simulink model "MPC_Quad_4SV"  (R2022b)
settings: Solver=FixedStepAuto  StartTime=0.0  StopTime=250  FixedStep=Ts  RelTol=1e-3
undefined symbols (not defined in the file): A, B, C, Cm, Ct, D, estim_hover_nrpm, g, initState, Ir, Ixx, Iyy, Izz, Length, mass
libraries: sharedtransform x5, uavutilslib x2, mpclib x1, shared6dof x1, aerolibutil x1
settings Model: PacingRate=0.005000  Creator=Bw Jiang  LastModifiedBy=Bw Jiang
settings DebuggingCC: AlgebraicLoopMsg=none  ParameterOverflowMsg=none  ParameterUnderflowMsg=error

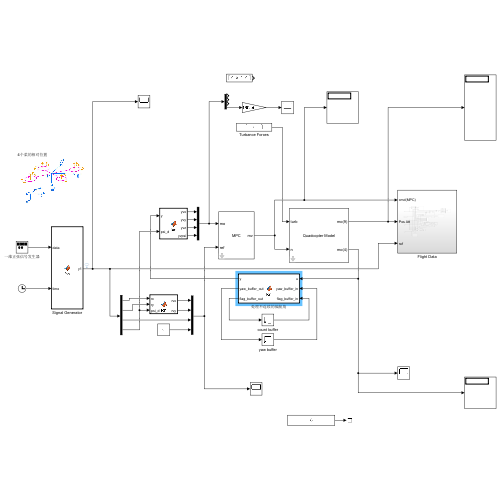
[thumbnail: Simulink's stored preview of the top-level diagram]
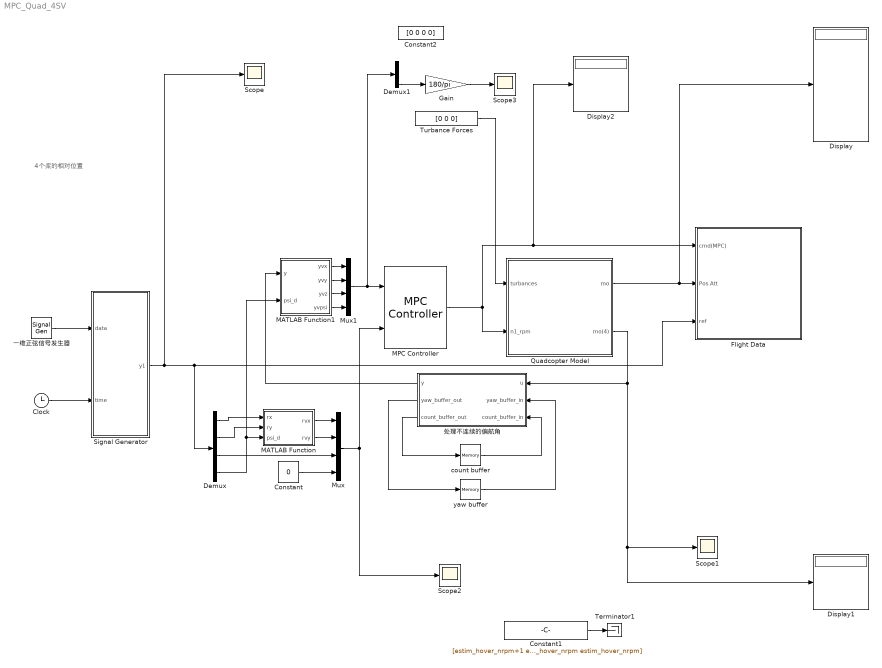
== system MPC_Quad_4SV ==
  note: 4个桨的相对位置
  Clock : Clock
  Constant : Constant  Value=0
  Constant1 : Constant  Value=[estim_hover_nrpm+1 estim_hover_nrpm estim_hover_nrpm estim_hover_nrpm]
  Constant2 : Constant  Value=[0 0 0 0]
  Demux : Demux
  Demux1 : Demux
  Display : Display
  Display1 : Display
  Display2 : Display
  Flight Data : Subsystem
  Gain : Gain  Gain=180/pi
  MATLAB Function : MATLAB Function  TreatAsAtomicUnit=on
  MATLAB Function1 : MATLAB Function  TreatAsAtomicUnit=on
  MPC Controller : mpclib/MPC Controller  SCDEnableBlockLinearizationSpecification=on  mpcobj=mpc4sv  is_multiple=0  enable_value=0  return_u0=off  updateMPCinCallerWorkspace=on  md_inport=off  mv_inport=off  uref_inport=off  return_cost=off  return_mvseq=off  return_qpstatus=off  return_xseq=off  return_state=off  return_ovseq=off  state_inport=off  umin_inport=off  umax_inport=off  ymin_inport=off  ymax_inport=off  cc_inport=off  ywt_inport=off  uwt_inport=off  duwt_inport=off  rhoeps_inport=off  pm_inport=off  MaximumP=10  HorizonChoice=FixedHorizon  n_ts=0.05  n_p=30  n_mv=4  n_md=0  n_ud=0  n_mo=4  n_uo=0  BlockDataType=double  SampleTimeInherited=off  switch_inport=off
  Mux : Mux
  Mux1 : Mux
  Quadcopter Model : Subsystem  mask{g=g, mass=mass, I_xx=Ixx, I_yy=Iyy, I_zz=Izz, I_r=Ir, L=Length, C_M=Cm, C_T=Ct}
      mask prompts: g "Gravity"; I_xx "Inertia_xx"; I_yy "Inertia_yy"; I_zz "Inertia_zz"; I_r "Inertia_per_rotor"; L "Length"
      mask DialogControl ParameterGroupVar Prompt: 参数
      mask Display:
      | disp('Quadcopter Model');
      | port_label('input', 1, 'turb')
      | port_label('input', 2, 'n')
      | % port_label('input', 3, 'n3')
      | % port_label('input', 4, 'n4')
      | port_label('output', 1, 'mo(9)')
      | port_label('output', 2, 'mo(4)')
      | % port_label('output', 3, 'y')
      | % port_label('output', 4, 'vy')
      | % port_label('output', 5, 'z')
      | % port_label('output', 6, 'vz')
      | % port_label('output', 7, 'phi')
      | % port_label('output', 8, 'd_phi')
      | % port_label('output', 9, 'theta')
      | % port_label('output', 10, 'd_theta')
      | % port_label('output', 11, 'psi')
      | % port_label('output', 12, 'd_psi')
  Scope{,1..3} (4 alike) : Scope
  Signal Generator : MATLAB Function  TreatAsAtomicUnit=on
  Terminator1 : Terminator
  Turbance Forces : Constant  Value=[0 0 0]
  count buffer : Memory
  yaw buffer : Memory
  一维正弦信号发生器 : SignalGenerator  Frequency=0.01
  处理不连续的偏航角 : MATLAB Function  TreatAsAtomicUnit=on
  wires:
  Clock/1 -> Signal Generator/2(time)
  MPC Controller/1 -> Display2/1, Flight Data/1(cmd(MPC)), Quadcopter Model/2(n1_rpm)
  Constant1/1 -> Terminator1/1
  Quadcopter Model/1(mo) -> Display/1, Flight Data/2(Pos Att)
  Quadcopter Model/2(mo(4)) -> Display1/1, Scope1/1, 处理不连续的偏航角/1(u)
  一维正弦信号发生器/1 -> Signal Generator/1(data)
  Turbance Forces/1 -> Quadcopter Model/1(turbances)
  Signal Generator/1(y1) -> Flight Data/3(ref), Demux/1, Scope/1
  Demux/3 -> Mux/3
  Constant/1 -> Mux/4
  Demux/1 -> MATLAB Function/1(rx)
  Demux/2 -> MATLAB Function/2(ry)
  Demux/4 -> MATLAB Function1/2(psi_d), MATLAB Function/3(psi_d)
  MATLAB Function/1(rvx) -> Mux/1
  MATLAB Function/2(rvy) -> Mux/2
  Mux/1 -> MPC Controller/2, Scope2/1
  MATLAB Function1/1(yvx) -> Mux1/1
  MATLAB Function1/2(yvy) -> Mux1/2
  MATLAB Function1/3(yvz) -> Mux1/3
  MATLAB Function1/4(yvpsi) -> Mux1/4
  Mux1/1 -> Demux1/1, MPC Controller/1
  Demux1/4 -> Gain/1
  Gain/1 -> Scope3/1
  处理不连续的偏航角/2(yaw_buffer_out) -> yaw buffer/1
  yaw buffer/1 -> 处理不连续的偏航角/2(yaw_buffer_in)
  count buffer/1 -> 处理不连续的偏航角/3(count_buffer_in)
  处理不连续的偏航角/3(count_buffer_out) -> count buffer/1
  处理不连续的偏航角/1(y) -> MATLAB Function1/1(y)

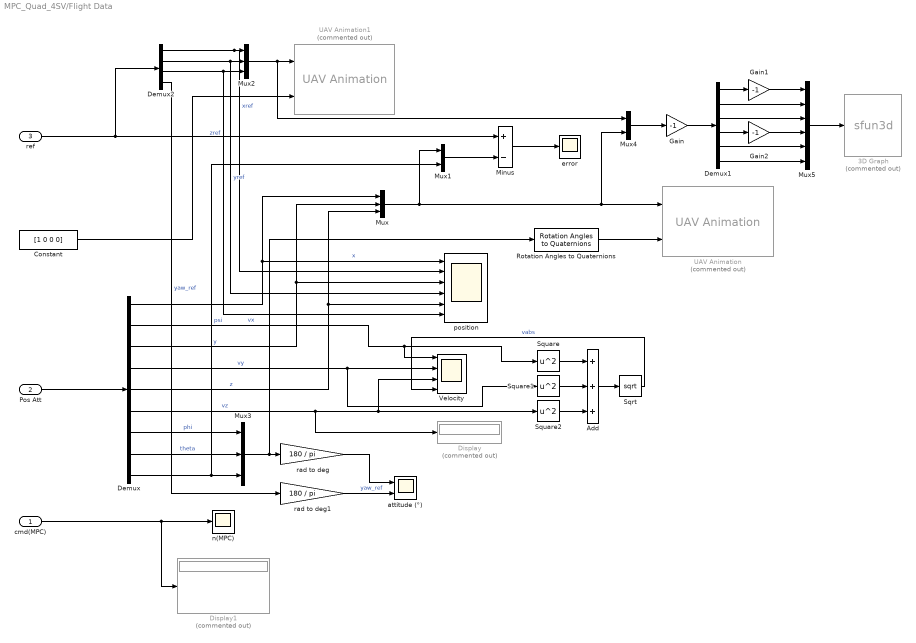
== system MPC_Quad_4SV/Flight Data ==
  cmd(MPC) : Inport
  Pos Att : Inport  Port=2
  ref : Inport  Port=3
  3D Graph : S-Function  Commented=on  LoadFcn=if exist('sfun3d','file'), sfun3d([],[],[],'LoadBlock'); end  FunctionName=sfun3d  Parameters=ax,T,np,cp,gd,ls,mk,mx,hd,tb  SFunctionDeploymentMode=off  EnableBusSupport=off  mask(3D Graph){np=2, ax=[-20 10 -10 10 -20 5], mx=50000, T=0.1, cp=[20 40 30], gd=on, hd=on, tb=on, ls=-, mk=none}
      mask prompts: np "Number of moving points (lines)"; ax "Range: [xmin xmax  ymin ymax zmin zmax]"; mx "Max number of points in each line"; T "Sampling Time"; cp "Camera position (use [0 0 1] for 2D XY view)"; gd "Grid (on|off)"; hd "HeadMarkers (on|off)"; tb "Toolbar (on|off)"; ls "LineStyle"; mk "LineMarker"
      mask help:
      | This block plots the position of several points in the XYZ space. The input contains the coordinates of all the points (x1,y1,z1,x2,y2,z2,...).
      | The number of moving points (lines), the XYZ ranges, sampling time, camera position, and grid (among other things) can be set as mask parameters.
      settings: CopyFcn=if exist('sfun3d','file'), sfun3d([],[],[],'CopyBlock'); end  DeleteFcn=if exist('sfun3d','file'), sfun3d([],[],[],'DeleteBlock'); end  NameChangeFcn=if exist('sfun3d','file'), sfun3d([],[],[],'NameChange'); end
      mask Help:
      | This block plots the position of several points in the XYZ space. The input contains the coordinates of all the points (x1,y1,z1,x2,y2,z2,...).
      | The number of moving points (lines), the XYZ ranges, sampling time, camera position, and grid (among other things) can be set as mask parameters.
      mask TypeOptions ls: - | -- | : | -. | none
      mask TypeOptions mk: none | . | + | o | * | x | square | diamond | v | ^ | > | < | pentagram | hexagram
      mask Display: plot([.05 .95 .95 .05 .05],[.45 .45 .95 .95 .45], 0.5+cos(0:0.1:2*pi)*0.3,0.7+sin(0:0.1:2*pi)*0.2)
  Add : Sum  Inputs=+++
  Constant : Constant  Value=[1 0 0 0]
  Demux : Demux  Outputs=9
  Demux1 : Demux  Outputs=6
  Demux2 : Demux
  Display : Display  Commented=on
  Display1 : Display  Commented=on
  Gain : Gain  Gain=-1
  Gain1 : Gain  Gain=-1
  Gain2 : Gain  Gain=-1
  Minus : Sum  Inputs=+-
  Mux : Mux  Inputs=3
  Mux1 : Mux  Inputs=2
  Mux2 : Mux  Inputs=3
  Mux3 : Mux  Inputs=3
  Mux4 : Mux  Inputs=2
  Mux5 : Mux  Inputs=6
  Rotation Angles to Quaternions : sharedtransform/Rotation Angles to Quaternions  rotationOrder=XYZ  aMode=aMode
  Sqrt : Sqrt
  Square : Math  Operator=square
  Square1 : Math  Operator=square
  Square2 : Math  Operator=square
  UAV Animation : uavutilslib/UAV Animation  Commented=on  UAVType=Multirotor  UAVSize=1  InertialZDirection=Down  SampleTime=-1
  UAV Animation1 : uavutilslib/UAV Animation  Commented=on  UAVType=Multirotor  UAVSize=1  InertialZDirection=Down  SampleTime=-1
  Velocity : Scope  NumInputPorts=4
  attitude (°) : Scope  NumInputPorts=2
  error : Scope
  n(MPC) : Scope
  position : Scope  NumInputPorts=6
  rad to deg : Gain  Gain=180 / pi
  rad to deg1 : Gain  Gain=180 / pi
  wires:
  Demux/8 -> Mux3/2  "theta"
  Demux/4 -> Square1/1, Velocity/2  "vy"
  Demux/2 -> Velocity/1, Square/1  "vx"
  Demux/7 -> Mux3/1  "phi"
  Demux/6 -> Velocity/3, Square2/1, Display/1  "vz"
  Demux/5 -> Mux/3, position/5  "z"
  Demux/1 -> Mux/1, position/1  "x"
  Demux/3 -> position/3, Mux/2  "y"
  rad to deg/1 -> attitude (°)/1
  Mux3/1 -> Rotation Angles to Quaternions/1, rad to deg/1
  cmd(MPC)/1 -> n(MPC)/1, Display1/1
  Pos Att/1 -> Demux/1
  Demux/9 -> Mux1/2, Mux3/3  "psi"
  Mux/1 -> Mux4/2, UAV Animation/1, Mux1/1
  Constant/1 -> UAV Animation1/2
  Mux1/1 -> Minus/2
  Minus/1 -> error/1
  ref/1 -> Demux2/1, Minus/1
  Demux2/1 -> position/2, Mux2/1  "xref"
  Demux2/2 -> position/4, Mux2/2  "yref"
  Demux2/3 -> position/6, Mux2/3  "zref"
  Mux2/1 -> Mux4/1, UAV Animation1/1
  Square/1 -> Add/1
  Square1/1 -> Add/2
  Square2/1 -> Add/3
  Add/1 -> Sqrt/1
  Sqrt/1 -> Velocity/4  "vabs"
  Mux4/1 -> Gain/1
  Gain/1 -> Demux1/1
  Demux1/1 -> Gain1/1
  Demux1/4 -> Gain2/1
  Gain1/1 -> Mux5/1
  Demux1/2 -> Mux5/2
  Demux1/3 -> Mux5/3
  Gain2/1 -> Mux5/4
  Demux1/5 -> Mux5/5
  Demux1/6 -> Mux5/6
  Mux5/1 -> 3D Graph/1
  Demux2/4 -> rad to deg1/1  "yaw_ref"
  rad to deg1/1 -> attitude (°)/2  "yaw_ref"
  Rotation Angles to Quaternions/1 -> UAV Animation/2

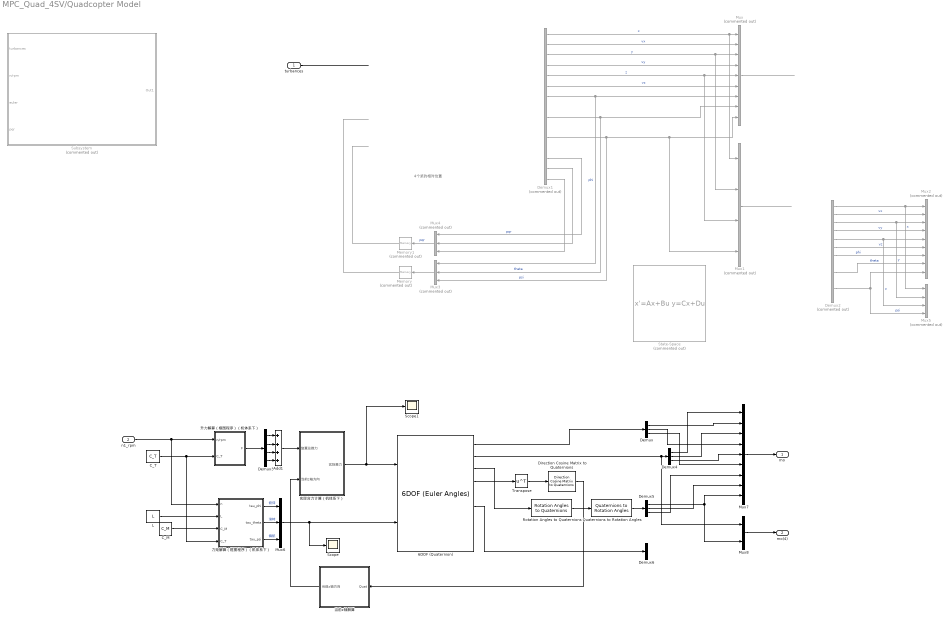
== system MPC_Quad_4SV/Quadcopter Model ==
  note: 4个桨的相对位置
  turbances : Inport
  n1_rpm : Inport  Port=2
  6DOF (Quaternion) : shared6dof/6DOF (Euler Angles)  units=Metric (MKS)  mtype=Fixed  rep=Euler Angles  xme_0=[initState.x, initState.y, initState.z]  Vm_0=[initState.vx, initState.vy, initState.vz]  eul_0=[initState.phi, initState.theta, initState.psi]  pm_0=[initState.p, initState.q, initState.r]  mass_0=mass  mass_e=0.5  mass_f=2.0  inertia=[Ixx, 0, 0; 0, Iyy, 0; 0, 0, Izz]  inertia_e=eye(3)  inertia_f=2*eye(3)  k_quat=Vehicle.SixDOF.quatGain  vre_flag=on  abi_flag=on  aMode=aMode  xme_statename=''  Vm_statename=''  eul_statename=''  quat_statename=''  pm_statename=''  mass_statename=''
  Add1 : Sum  Inputs=++++
  C_M : Constant  Value=C_M
  C_T : Constant  Value=C_T
  Demux{,4..6} (4 alike) : Demux  Outputs=3
  Demux1 : Demux  Commented=on  Outputs=15
  Demux2 : Demux  Commented=on  Outputs=12
  Demux3 : Demux
  Direction Cosine Matrix to Quaternions : sharedtransform/Direction Cosine Matrix  to Quaternions  aMode=0  action=None  tolerance=eps(2)
  L : Constant  Value=L
  Memory : Memory  Commented=on  InheritSampleTime=on
  Memory1 : Memory  Commented=on  InheritSampleTime=on
  Mux : Mux  Commented=on  Inputs=9
  Mux1 : Mux  Commented=on
  Mux2 : Mux  Commented=on  Inputs=9
  Mux3 : Mux  Commented=on  Inputs=3
  Mux4 : Mux  Commented=on  Inputs=3
  Mux5 : Mux  Commented=on
  Mux6 : Mux  Inputs=3
  Mux7 : Mux  Inputs=9
  Mux8 : Mux  Inputs=2
  Quaternions to Rotation Angles : sharedtransform/Quaternions to Rotation Angles  rotationOrder=XYZ  aMode=aMode
  Rotation Angles to Quaternions : sharedtransform/Rotation Angles to Quaternions  rotationOrder=ZYX  aMode=aMode
  Scope : Scope
  Scope1 : Scope
  State-Space : StateSpace  Commented=on  A=A  B=B  C=C  D=D  InitialCondition=0
  Subsystem : Subsystem  Commented=on
  Transpose : Math  Operator=transpose
  力矩解算（框图程序）（机体系下） : Subsystem
  升力解算（框图程序）（机体系下） : Subsystem
  实际合力计算（机体系下） : Subsystem
  当前z轴解算 : Subsystem
  mo : Outport
  mo(4) : Outport  Port=2
  wires:
  Memory1/1 -> ?
  Demux1/15 -> Mux4/3
  Demux1/13 -> Mux4/1  "pqr"
  Mux4/1 -> Memory1/1  "pqr"
  Demux1/9 -> Mux/8, Mux3/2  "theta"
  Demux1/1 -> Mux1/1, Mux/1  "x"
  Demux1/2 -> Mux/2  "vx"
  Demux1/11 -> Mux1/4, Mux/9, Mux3/3  "psi"
  Demux1/4 -> Mux/4  "vy"
  Demux1/3 -> Mux1/2, Mux/3  "y"
  Demux1/5 -> Mux1/3, Mux/5  "z"
  ? -> Demux1/1
  Memory/1 -> ?
  Demux1/6 -> Mux/6  "vz"
  Demux1/7 -> Mux/7, Mux3/1  "phi"
  Mux3/1 -> Memory/1
  Demux1/14 -> Mux4/2
  turbances/1 -> ?
  Demux2/1 -> Mux2/1, Mux5/1  "x"
  Demux2/2 -> Mux2/2  "vx"
  Demux2/3 -> Mux5/2, Mux2/3  "y"
  Demux2/4 -> Mux2/4  "vy"
  Demux2/5 -> Mux5/3, Mux2/5  "z"
  Demux2/6 -> Mux2/6  "vz"
  Demux2/7 -> Mux2/7  "phi"
  Demux2/9 -> Mux2/8  "theta"
  Demux2/11 -> Mux5/4, Mux2/9  "psi"
  Mux/1 -> ?
  Mux1/1 -> ?
  n1_rpm/1 -> 力矩解算（框图程序）（机体系下）/1(n), 升力解算（框图程序）（机体系下）/1(n/rpm)
  力矩解算（框图程序）（机体系下）/3(tau_psi) -> Mux6/3  "偏航"
  实际合力计算（机体系下）/1(实际推力) -> Scope1/1, 6DOF (Quaternion)/1
  力矩解算（框图程序）（机体系下）/2(tau_theta) -> Mux6/2  "滚转"
  L/1 -> 力矩解算（框图程序）（机体系下）/2(L)
  Rotation Angles to Quaternions/1 -> Quaternions to Rotation Angles/1
  6DOF (Quaternion)/1 -> Demux/1
  6DOF (Quaternion)/3 -> Rotation Angles to Quaternions/1
  C_M/1 -> 力矩解算（框图程序）（机体系下）/3(C_M)
  Demux3/1 -> Add1/1
  Quaternions to Rotation Angles/1 -> Demux5/1
  Mux6/1 -> Scope/1, 6DOF (Quaternion)/2
  6DOF (Quaternion)/2 -> Mux8/1, Demux4/1
  Demux3/3 -> Add1/3
  当前z轴解算/1(当前z轴方向) -> 实际合力计算（机体系下）/2(当前z轴方向)
  升力解算（框图程序）（机体系下）/1(F) -> Demux3/1
  6DOF (Quaternion)/6 -> Demux6/1
  6DOF (Quaternion)/4 -> Transpose/1
  Demux3/4 -> Add1/4
  Direction Cosine Matrix to Quaternions/1 -> 当前z轴解算/1(Quat)
  Transpose/1 -> Direction Cosine Matrix to Quaternions/1
  C_T/1 -> 力矩解算（框图程序）（机体系下）/4(C_T), 升力解算（框图程序）（机体系下）/2(C_T)
  Demux3/2 -> Add1/2
  力矩解算（框图程序）（机体系下）/1(tau_phi) -> Mux6/1  "俯仰"
  Add1/1 -> 实际合力计算（机体系下）/1(旋翼总推力)
  Demux4/1 -> Mux7/1
  Demux/1 -> Mux7/2
  Demux4/2 -> Mux7/3
  Demux4/3 -> Mux7/5
  Demux/2 -> Mux7/4
  Demux/3 -> Mux7/6
  Demux5/1 -> Mux7/9, Mux8/2
  Demux5/2 -> Mux7/8
  Demux5/3 -> Mux7/7
  Mux7/1 -> mo/1
  Mux8/1 -> mo(4)/1

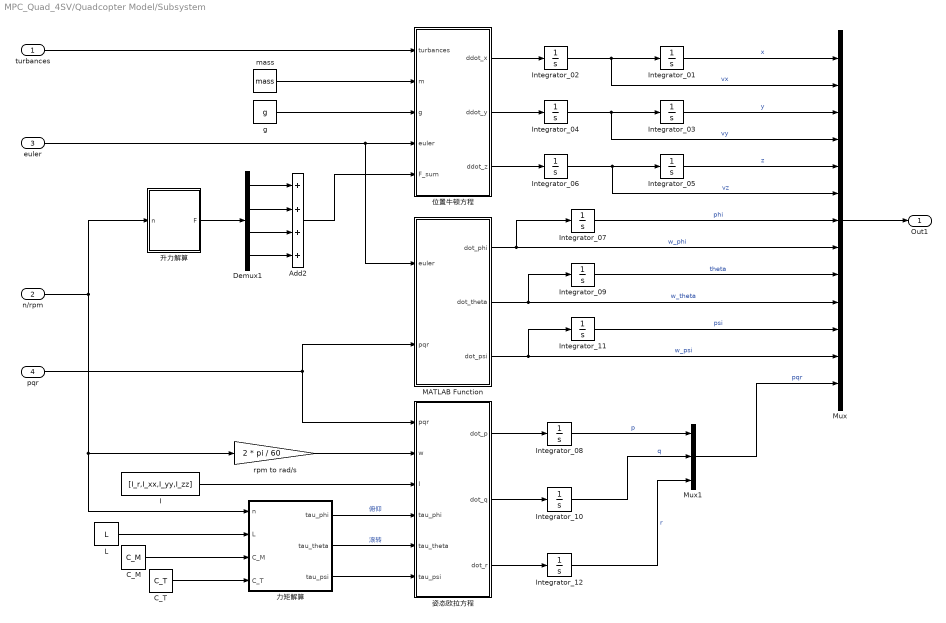
== system MPC_Quad_4SV/Quadcopter Model/Subsystem ==
  turbances : Inport
  n/rpm : Inport  Port=2  PortDimensions=4
  euler : Inport  Port=3  PortDimensions=3
  pqr : Inport  Port=4  PortDimensions=3
  Add2 : Sum  Inputs=++++
  C_M : Constant  Value=C_M
  C_T : Constant  Value=C_T
  Demux1 : Demux
  I : Constant  Value=[I_r,I_xx,I_yy,I_zz]
  Integrator_01 : Integrator  InitialCondition=initState.x
  Integrator_02 : Integrator  InitialCondition=initState.vx
  Integrator_03 : Integrator  InitialCondition=initState.y
  Integrator_04 : Integrator  InitialCondition=initState.vy
  Integrator_05 : Integrator  InitialCondition=initState.z
  Integrator_06 : Integrator  InitialCondition=initState.vz
  Integrator_07 : Integrator  InitialCondition=initState.phi
  Integrator_08 : Integrator  InitialCondition=initState.p
  Integrator_09 : Integrator  InitialCondition=initState.theta
  Integrator_10 : Integrator  InitialCondition=initState.q
  Integrator_11 : Integrator  InitialCondition=initState.psi
  Integrator_12 : Integrator  InitialCondition=initState.r
  L : Constant  Value=L
  MATLAB Function : MATLAB Function  TreatAsAtomicUnit=on
  Mux : Mux  Inputs=13
  Mux1 : Mux  Inputs=3
  g : Constant  Value=g
  mass : Constant  Value=mass
  rpm to rad/s : Gain  Gain=2 * pi / 60
  位置牛顿方程 : MATLAB Function  TreatAsAtomicUnit=on
  力矩解算 : MATLAB Function  TreatAsAtomicUnit=on
  升力解算 : MATLAB Function  TreatAsAtomicUnit=on
  姿态欧拉方程 : MATLAB Function  TreatAsAtomicUnit=on
  Out1 : Outport
  wires:
  姿态欧拉方程/1(dot_p) -> Integrator_08/1
  Demux1/4 -> Add2/4
  pqr/1 -> MATLAB Function/2(pqr), 姿态欧拉方程/1(pqr)
  位置牛顿方程/2(ddot_y) -> Integrator_04/1
  姿态欧拉方程/2(dot_q) -> Integrator_10/1
  I/1 -> 姿态欧拉方程/3(I)
  位置牛顿方程/3(ddot_z) -> Integrator_06/1
  Mux/1 -> Out1/1
  g/1 -> 位置牛顿方程/3(g)
  位置牛顿方程/1(ddot_x) -> Integrator_02/1
  Integrator_10/1 -> Mux1/2  "q"
  Demux1/1 -> Add2/1
  力矩解算/1(tau_phi) -> 姿态欧拉方程/4(tau_phi)  "俯仰"
  Integrator_08/1 -> Mux1/1  "p"
  euler/1 -> MATLAB Function/1(euler), 位置牛顿方程/4(euler)
  Integrator_03/1 -> Mux/3  "y"
  Integrator_09/1 -> Mux/9  "theta"
  力矩解算/3(tau_psi) -> 姿态欧拉方程/6(tau_psi)
  Demux1/2 -> Add2/2
  Add2/1 -> 位置牛顿方程/5(F_sum)
  Integrator_12/1 -> Mux1/3  "r"
  mass/1 -> 位置牛顿方程/2(m)
  力矩解算/2(tau_theta) -> 姿态欧拉方程/5(tau_theta)  "滚转"
  Demux1/3 -> Add2/3
  Integrator_05/1 -> Mux/5  "z"
  Integrator_01/1 -> Mux/1  "x"
  Integrator_02/1 -> Integrator_01/1, Mux/2  "vx"
  Integrator_07/1 -> Mux/7  "phi"
  Integrator_04/1 -> Mux/4, Integrator_03/1  "vy"
  Integrator_06/1 -> Mux/6, Integrator_05/1  "vz"
  Integrator_11/1 -> Mux/11  "psi"
  姿态欧拉方程/3(dot_r) -> Integrator_12/1
  MATLAB Function/3(dot_psi) -> Integrator_11/1, Mux/12  "w_psi"
  MATLAB Function/2(dot_theta) -> Integrator_09/1, Mux/10  "w_theta"
  MATLAB Function/1(dot_phi) -> Integrator_07/1, Mux/8  "w_phi"
  Mux1/1 -> Mux/13  "pqr"
  升力解算/1(F) -> Demux1/1
  L/1 -> 力矩解算/2(L)
  n/rpm/1 -> 升力解算/1(n), rpm to rad/s/1, 力矩解算/1(n)
  rpm to rad/s/1 -> 姿态欧拉方程/2(w)
  C_M/1 -> 力矩解算/3(C_M)
  C_T/1 -> 力矩解算/4(C_T)
  turbances/1 -> 位置牛顿方程/1(turbances)

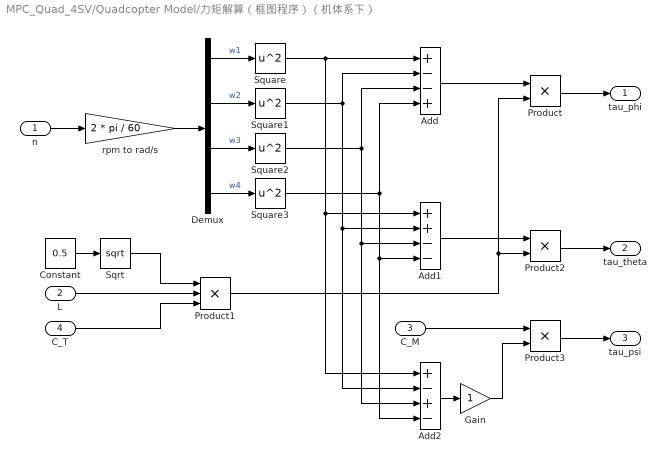
== system MPC_Quad_4SV/Quadcopter Model/力矩解算（框图程序）（机体系下） ==
  n : Inport
  L : Inport  Port=2
  C_M : Inport  Port=3
  C_T : Inport  Port=4
  Add : Sum  Inputs=+--+
  Add1 : Sum  Inputs=++--
  Add2 : Sum  Inputs=+-+-
  Constant : Constant  Value=0.5
  Demux : Demux
  Gain : Gain
  Product : Product
  Product1 : Product  Inputs=3
  Product2 : Product
  Product3 : Product
  Sqrt : Sqrt
  Square{,1..3} (4 alike) : Math  Operator=square
  rpm to rad/s : Gain  Gain=2 * pi / 60
  tau_phi : Outport
  tau_theta : Outport  Port=2
  tau_psi : Outport  Port=3
  wires:
  rpm to rad/s/1 -> Demux/1
  n/1 -> rpm to rad/s/1
  Demux/1 -> Square/1  "w1"
  Demux/2 -> Square1/1  "w2"
  Demux/3 -> Square2/1  "w3"
  Demux/4 -> Square3/1  "w4"
  Square/1 -> Add1/1, Add2/1, Add/1
  Square1/1 -> Add1/2, Add2/2, Add/2
  Square2/1 -> Add2/3, Add1/3, Add/3
  Square3/1 -> Add2/4, Add1/4, Add/4
  Add/1 -> Product/1
  L/1 -> Product1/2
  C_T/1 -> Product1/3
  Constant/1 -> Sqrt/1
  Sqrt/1 -> Product1/1
  Product1/1 -> Product/2, Product2/2
  Product/1 -> tau_phi/1
  Add1/1 -> Product2/1
  Product2/1 -> tau_theta/1
  Add2/1 -> Gain/1
  C_M/1 -> Product3/1
  Product3/1 -> tau_psi/1
  Gain/1 -> Product3/2

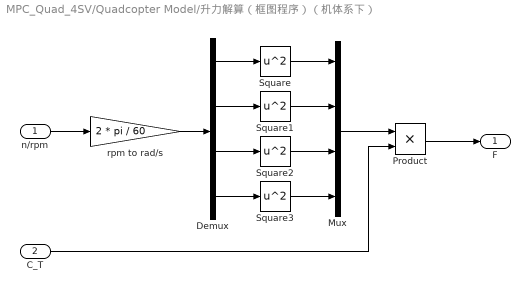
== system MPC_Quad_4SV/Quadcopter Model/升力解算（框图程序）（机体系下） ==
  n/rpm : Inport
  C_T : Inport  Port=2
  Demux : Demux
  Mux : Mux
  Product : Product
  Square{,1..3} (4 alike) : Math  Operator=square
  rpm to rad/s : Gain  Gain=2 * pi / 60
  F : Outport
  wires:
  n/rpm/1 -> rpm to rad/s/1
  rpm to rad/s/1 -> Demux/1
  Demux/1 -> Square/1
  Demux/2 -> Square1/1
  Demux/3 -> Square2/1
  Demux/4 -> Square3/1
  Square3/1 -> Mux/4
  Square2/1 -> Mux/3
  Square1/1 -> Mux/2
  Square/1 -> Mux/1
  Mux/1 -> Product/1
  C_T/1 -> Product/2
  Product/1 -> F/1

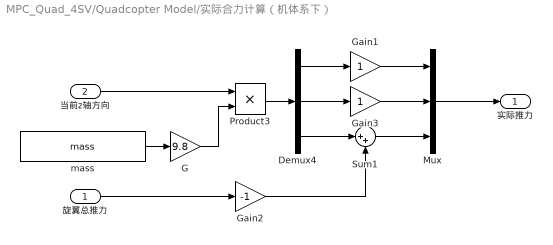
== system MPC_Quad_4SV/Quadcopter Model/实际合力计算（机体系下） ==
  旋翼总推力 : Inport
  当前z轴方向 : Inport  Port=2
  Demux4 : Demux  Outputs=3
  G : Gain  Gain=9.8
  Gain1 : Gain
  Gain2 : Gain  Gain=-1
  Gain3 : Gain
  Mux : Mux  Inputs=3
  Product3 : Product
  Sum1 : Sum  Inputs=|++
  mass : Constant  Value=mass
  实际推力 : Outport
  wires:
  Demux4/1 -> Gain1/1
  当前z轴方向/1 -> Product3/1
  G/1 -> Product3/2
  Sum1/1 -> Mux/3
  Demux4/2 -> Gain3/1
  mass/1 -> G/1
  Product3/1 -> Demux4/1
  Mux/1 -> 实际推力/1
  旋翼总推力/1 -> Gain2/1
  Gain1/1 -> Mux/1
  Gain3/1 -> Mux/2
  Demux4/3 -> Sum1/1
  Gain2/1 -> Sum1/2

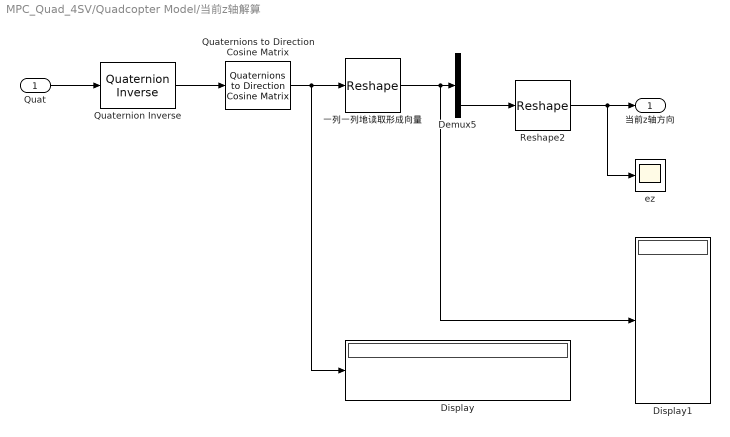
== system MPC_Quad_4SV/Quadcopter Model/当前z轴解算 ==
  Quat : Inport
  Demux5 : Demux  Outputs=3
  Display : Display
  Display1 : Display
  Quaternion Inverse : aerolibutil/Quaternion Inverse
  Quaternions to Direction Cosine Matrix : sharedtransform/Quaternions to  Direction Cosine Matrix  aMode=aMode
  Reshape2 : Reshape  OutputDimensionality=Row vector (2-D)
  ez : Scope
  一列一列地读取形成向量 : Reshape  OutputDimensionality=Column vector (2-D)
  当前z轴方向 : Outport
  wires:
  Quat/1 -> Quaternion Inverse/1
  Demux5/3 -> Reshape2/1
  Reshape2/1 -> 当前z轴方向/1, ez/1
  Quaternions to Direction Cosine Matrix/1 -> Display/1, 一列一列地读取形成向量/1
  一列一列地读取形成向量/1 -> Display1/1, Demux5/1
  Quaternion Inverse/1 -> Quaternions to Direction Cosine Matrix/1

== matlab function MPC_Quad_4SV/处理不连续的偏航角 ==
  data: u input; y output; yaw_buffer_in input; yaw_buffer_out output; count_buffer_in input; count_buffer_out output
function [y, yaw_buffer_out, count_buffer_out] = fcn(u, yaw_buffer_in, count_buffer_in)

% 处理不连续的偏航角
% 因为物理模块输出的yaw在(-pi, pi]之间
% 该模块的意义在于将提供给MPC的yaw放大到(-inf, +inf)
% 当检测到越过±pi时就相应地加上或减去一个周期，加一个周期称为正向越过，反之为逆向越过
% 角度均为弧度制
% yaw buffer保存前一个分析步的yaw，其值位于(-pi, pi]，用于与当前时间步对比，判断是否发生越过
% count buffer保存总共正向越过几次，正向越过一次+1，逆向越过一次-1

yaw = u(4);
count = count_buffer_in;
delta_count = 0;
yaw_buffer_out = u(4);

if yaw_buffer_in >= 150 * pi / 180
    if yaw < 0
        delta_count = 1;
    end
end

if yaw_buffer_in <= -150 * pi / 180
    if yaw > 0
        delta_count = -1;
    end
end

count = count + delta_count;

u(4) = u(4) + count * 2 * pi;

count_buffer_out = count;

y = u;

end

== matlab function MPC_Quad_4SV/Quadcopter Model/Subsystem/MATLAB Function ==
  data: euler input; pqr input; dot_phi output; dot_theta output; dot_psi output
function [dot_phi, dot_theta, dot_psi] = fcn(euler, pqr)

% 角加速度的坐标转换，从机体系b到惯性系e

p = pqr(1);
q = pqr(2);
r = pqr(3);

phi =euler(1);
theta = euler(2);
psi = euler(3);

mat = [
    1, tan(theta) * sin(phi), tan(theta) * cos(phi);
    0, cos(phi), -sin(phi);
    0, sin(phi) / cos(theta), cos(phi) / cos(theta)
    ];
body = [p; q; r];
earth = mat * body;

dot_phi = earth(1);
dot_theta = earth(2);
dot_psi = earth(3);

== matlab function MPC_Quad_4SV/Quadcopter Model/Subsystem/位置牛顿方程 ==
  data: turbances input; m input; g input; euler input; ddot_x output; F_sum input; ddot_y output; ddot_z output
function [ddot_x, ddot_y, ddot_z] = fcn(turbances, m, g, euler, F_sum)

% F_sum恒正

phi =euler(1);
theta = euler(2);
psi = euler(3);

ddot_x = -((cos(phi) * sin(theta) * cos(psi) + sin(phi) * sin(psi)) * F_sum + turbances(1)) / m;
ddot_y = -((cos(phi) * sin(theta) * sin(psi) - sin(phi) * cos(psi)) * F_sum + turbances(2)) / m;
ddot_z = -(cos(phi) * cos(theta) * F_sum + turbances(3)) / m + g;

end

== matlab function MPC_Quad_4SV/Quadcopter Model/Subsystem/姿态欧拉方程 ==
  data: pqr input; dot_p output; w input; I input; dot_q output; dot_r output; tau_phi input; tau_theta input; tau_psi input
function [dot_p, dot_q, dot_r] = fcn(pqr, w, I, tau_phi, tau_theta, tau_psi)

w1 = w(1);
w2 = w(2);
w3 = w(3);
w4 = w(4);

p = pqr(1);
q = pqr(2);
r = pqr(3);

I_r = I(1);
I_xx = I(2);
I_yy = I(3);
I_zz = I(4);

w_tau = w1 - w2 + w3 - w4;

dot_p = (I_yy - I_zz) / I_xx * q * r - I_r * q / I_xx * w_tau + tau_phi / I_xx;
dot_q = (I_zz - I_xx) / I_yy * p * r + I_r * p / I_yy * w_tau + tau_theta / I_yy;
dot_r = (I_xx - I_yy) / I_zz * q * p + tau_psi / I_zz;

end

== matlab function MPC_Quad_4SV/Quadcopter Model/Subsystem/升力解算 ==
  data: n input; F output
function F = fcn(n)
%% Input Vars
% n - rpm

%% Output Vars
% F - N

%% Mid Vars
% omega - rad/s

%% Code

% F = n .* n * 2.414e-7 * 2;

omega = n / 60 * 2 * pi;
F = omega .* omega * 1.11e-5;

end

== matlab function MPC_Quad_4SV/Signal Generator ==
  data: data input; time input; y1 output
function y1  = fcn(data, time)

starttime = 2;

%% 悬停

% y1 = [0
%       0
%       0
%       pi/2];

%% 螺旋线轨迹

% radspeed = 45; % 相当于相对圆心角的角速度 °/s
% vz = 0;
% r = 2 + time * 0.0;
% if time < starttime
%     y1 = [0
%           0
%           0
%           0];
% else
%     if r > 15
%         r = 15;
%     end
%     y1 = [r - r * cos(radspeed * (time - starttime) * pi / 180)
%           r * sin(radspeed * (time - starttime) * pi / 180)
%           -vz * time
%           0];
% end

%% 类8字轨迹

% radspeed = 10; % 相当于相对圆心角的角速度 °/s
% vz = 0.2;
% r1 = 4;
% r2 = 8;
% if time < starttime
%     y1 = [0; 0; 0; 0];
% else
%     if time < starttime + 180 / radspeed
%         y1 = [r1 - r1 * cos(radspeed * (time - starttime) * pi / 180)
%               r1 * sin(radspeed * (time - starttime) * pi / 180)
%               vz * (time - starttime)
%               0];
%     else
%         if time < starttime + 360 / radspeed
%             y1 = [-r2 * cos(radspeed * (time - starttime) * pi / 180)
%                   r2 * sin(radspeed * (time - starttime) * pi / 180)
%                   vz * (time - starttime)
%                   0];
%         else
%             if time < starttime + 540 / radspeed
%                 y1 = [-(r1 + r2) + r1 * cos(- radspeed * (time - starttime - 360 / radspeed) * pi / 180)
%                       r1 * sin(radspeed * (time - starttime) * pi / 180)
%                       vz * 360 / radspeed - vz * (time - starttime - 360 / radspeed)
%                       0];
%             else
%                 if time < starttime + 720 / radspeed
%                     y1 = [-r2 + r2 * cos(2 * pi - radspeed * (time - starttime - 360 / radspeed) * pi / 180)
%                           r2 * sin(radspeed * (time - starttime - 360 / radspeed) * pi / 180)
%                           vz * 360 / radspeed - vz * (time - starttime - 360 / radspeed)
%                           0];
%                 else
%                     y1 = [0; 0; 0; 0];
%                 end
%             end
%         end
%     end
% end

%% 阶跃轨迹

% x = 0;
% y = 0;
% z = 0;
% yaw = 0;
% 
% if time < 10
%     x = 0;
%     y = 0;
%     z = 0;
%     yaw = 0;
% elseif time > 10
%     x = 1;
%     y = 1.2;
%     z = -0.8;
%     yaw = 0;
% end
% 
% y1 = [x
%     y
%     z
%     yaw];

%% 偏航控制测试

yawspeed = 10; % °/s
yawspeed = yawspeed * pi / 180; % convert to rad/s

t1 = starttime + 3;
t2 = t1 + 30;
t3 = t2 + 100;
t4 = t3 + 50;
t5 = t4 + 30;
if time < starttime
    y1 = [0
          0
          0
          0];
else
    if time < t1
    y1 = [0
          0
          0
          yawspeed * (time - starttime)];
    else
        if time < t2
            y1 = [0
                  0
                  0
                  yawspeed * (t1 - starttime)];
        else
            if time < t3
                y1 = [0
                      0
                      0
                      yawspeed * (time - t2 + t1 - starttime)];
            else
                if time < t4
                    y1 = [0
                          0
                          0
                          yawspeed * (t3 - t2 + t1 - starttime)];

                else
                    if time < t5
                        y1 = [0
                              0
                              0
                              yawspeed * (t3 - t2 + t1 - starttime) / (t4 - t5) * (time - t5)];
                    else
                        y1 = [0
                              0
                              0
                              0];
                    end
                end
            end
        end
    end
end

end

== matlab function MPC_Quad_4SV/Quadcopter Model/Subsystem/力矩解算 ==
  data: n input; L input; tau_phi output; tau_theta output; tau_psi output; C_M input; C_T input
function [tau_phi, tau_theta, tau_psi]= fcn(n, L, C_M, C_T)
%% Input Vars
% n - rpm
% L - m
% C_M - N*m*s^2/rad^2
% C_T - N*s^2/rad^2

%% Output Vars
% tau - N*m

%% Mid Vars
% w - rad/s

%% Code

% C_T = 1.1e-5;
% C_M = 1.0144e-7;

% F1 = F(1);
% F2 = F(2);
% F3 = F(3);
% F4 = F(4);

w1 = n(1) / 60 * 2 * pi;
w2 = n(2) / 60 * 2 * pi;
w3 = n(3) / 60 * 2 * pi;
w4 = n(4) / 60 * 2 * pi;

% I_r = I(1);

% w_tau = w1 + w3 - w2 - w4;

% 横滚
tau_phi = sqrt(2) / 2 * C_T * L * (w1^2 - w2^2 - w3^2 + w4^2); % tau_phi = (F1+F2-F3-F4) * L;
% 俯仰
tau_theta = sqrt(2) / 2 * C_T * L * (w1^2 + w2^2 - w3^2 - w4^2); % tau_theta = (F1-F2-F3+F4) * L;
% 偏航
tau_psi = C_M * (w1^2 - w2^2 + w3^2 - w4^2); % tau_psi = w_tau * I_r;

end

== matlab function MPC_Quad_4SV/MATLAB Function ==
  data: rx input; rvx output; ry input; psi_d input; rvy output
function [rvx, rvy] = fcn(rx, ry, psi_d)

rvx = rx * cos(psi_d) + ry * sin(psi_d);
rvy = -rx * sin(psi_d) + ry * cos(psi_d);

end

== matlab function MPC_Quad_4SV/MATLAB Function1 ==
  data: y input; yvx output; psi_d input; yvy output; yvz output; yvpsi output
function [yvx, yvy, yvz, yvpsi] = fcn(y, psi_d)

yx = y(1);
yy = y(2);
yz = y(3);
ypsi = y(4);

yvx = yx * cos(psi_d) + yy * sin(psi_d);
yvy = -yx * sin(psi_d) + yy * cos(psi_d);
yvz = yz;
yvpsi = ypsi - psi_d;

end
